simulink model "validate_emotor_start_stop"  (R2015a)
settings: Solver=ode45  StartTime=0.0  StopTime=10.0  RelTol=1e-3
settings Model: Creator=Piyush  LastModifiedBy=Piyush

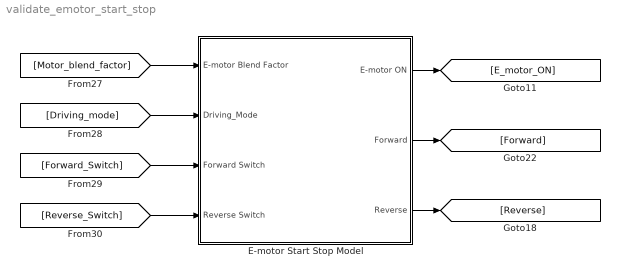
== system validate_emotor_start_stop ==
  E-motor Start Stop Model : Subsystem
  wires:
  [Motor_blend_factor] -> E-motor Start Stop Model/1(E-motor Blend Factor)
  [Driving_mode] -> E-motor Start Stop Model/2(Driving_Mode)
  [Forward_Switch] -> E-motor Start Stop Model/3(Forward Switch)
  [Reverse_Switch] -> E-motor Start Stop Model/4(Reverse Switch)
  E-motor Start Stop Model/3(Reverse) -> [Reverse]
  E-motor Start Stop Model/2(Forward) -> [Forward]
  E-motor Start Stop Model/1(E-motor ON) -> [E_motor_ON]

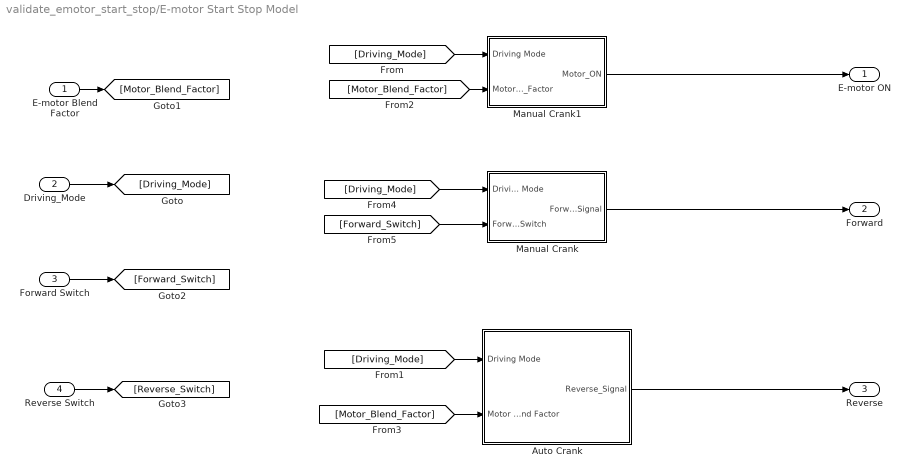
== system validate_emotor_start_stop/E-motor Start Stop Model ==
  E-motor Blend Factor : Inport
  Driving_Mode : Inport  Port=2
  Forward Switch : Inport  Port=3
  Reverse Switch : Inport  Port=4
  Auto Crank : Subsystem
  Manual Crank : Subsystem
  Manual Crank1 : Subsystem
  E-motor ON : Outport
  Forward : Outport  Port=2
  Reverse : Outport  Port=3
  wires:
  [Forward_Switch] -> Manual Crank/2(Forward Switch)
  Manual Crank1/1(Motor_ON) -> E-motor ON/1
  [Driving_Mode] -> Manual Crank1/1(Driving Mode)
  [Driving_Mode] -> Auto Crank/1(Driving Mode)
  [Motor_Blend_Factor] -> Manual Crank1/2(Motor_Blend_Factor)
  [Motor_Blend_Factor] -> Auto Crank/2(Motor Blend Factor)
  [Driving_Mode] -> Manual Crank/1(Driving Mode)
  E-motor Blend Factor/1 -> [Motor_Blend_Factor]
  Driving_Mode/1 -> [Driving_Mode]
  Forward Switch/1 -> [Forward_Switch]
  Reverse Switch/1 -> [Reverse_Switch]
  Auto Crank/1(Reverse_Signal) -> Reverse/1
  Manual Crank/1(Forward_Signal) -> Forward/1

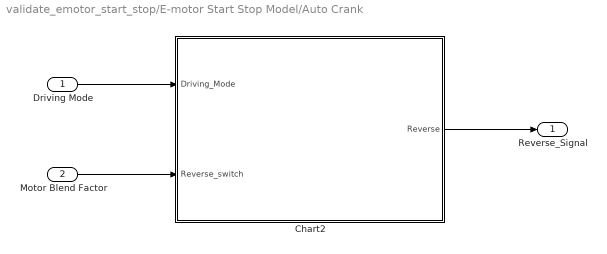
== system validate_emotor_start_stop/E-motor Start Stop Model/Auto Crank ==
  Driving Mode : Inport
  Motor Blend Factor : Inport  Port=2
  Chart2 : Stateflow chart  TreatAsAtomicUnit=on
  Reverse_Signal : Outport
  wires:
  Chart2/1(Reverse) -> Reverse_Signal/1
  Driving Mode/1 -> Chart2/1(Driving_Mode)
  Motor Blend Factor/1 -> Chart2/2(Reverse_switch)

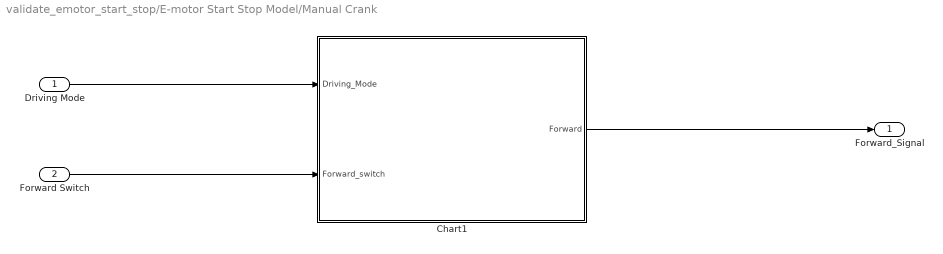
== system validate_emotor_start_stop/E-motor Start Stop Model/Manual Crank ==
  Driving Mode : Inport
  Forward Switch : Inport  Port=2
  Chart1 : Stateflow chart  TreatAsAtomicUnit=on
  Forward_Signal : Outport
  wires:
  Chart1/1(Forward) -> Forward_Signal/1
  Driving Mode/1 -> Chart1/1(Driving_Mode)
  Forward Switch/1 -> Chart1/2(Forward_switch)

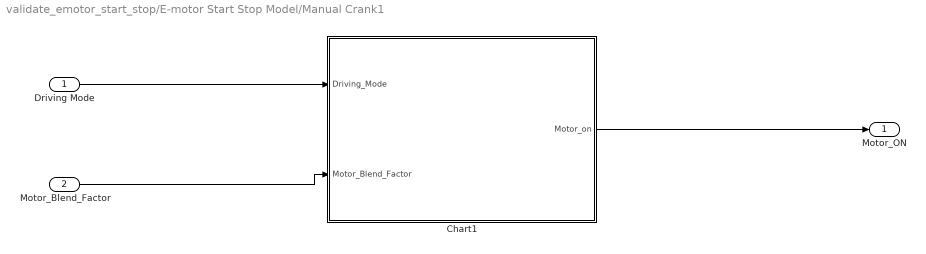
== system validate_emotor_start_stop/E-motor Start Stop Model/Manual Crank1 ==
  Driving Mode : Inport
  Motor_Blend_Factor : Inport  Port=2
  Chart1 : Stateflow chart  TreatAsAtomicUnit=on
  Motor_ON : Outport
  wires:
  Driving Mode/1 -> Chart1/1(Driving_Mode)
  Motor_Blend_Factor/1 -> Chart1/2(Motor_Blend_Factor)
  Chart1/1(Motor_on) -> Motor_ON/1

== stateflow chart validate_emotor_start_stop/E-motor Start Stop Model/Auto Crank/Chart2 ==
  state REVERSE_ON
    during: Reverse=1;
  state REVERSE_OFF
    during: Reverse=0;
  REVERSE_ON -> REVERSE_OFF : [Driving_Mode==2||Driving_Mode==3]
  REVERSE_OFF -> REVERSE_ON : [Driving_Mode==1&&Reverse_switch==1]
  (default) -> REVERSE_OFF
  data: Driving_Mode input; Reverse_switch input; Reverse output

== stateflow chart validate_emotor_start_stop/E-motor Start Stop Model/Manual Crank/Chart1 ==
  state FORWARD_ON
    during: Forward=1;
  state FORWARD_OFF
    during: Forward=0;
  FORWARD_ON -> FORWARD_OFF : [Driving_Mode==3]
  FORWARD_OFF -> FORWARD_ON [order 1] : [Driving_Mode==2]
  FORWARD_OFF -> FORWARD_ON [order 2] : [Driving_Mode==1&&Forward_switch==1]
  (default) -> FORWARD_OFF
  data: Driving_Mode input; Forward_switch input; Forward output

== stateflow chart validate_emotor_start_stop/E-motor Start Stop Model/Manual Crank1/Chart1 ==
  state MOTOR_ON
    during: Motor_on=1;
  state MOTOR_OFF
    during: Motor_on=0;
  MOTOR_ON -> MOTOR_OFF [order 2] : [Driving_Mode==2&&Motor_Blend_Factor<0.01]
  MOTOR_ON -> MOTOR_OFF [order 1] : [Driving_Mode==3]
  MOTOR_OFF -> MOTOR_ON [order 1] : [Driving_Mode==1]
  MOTOR_OFF -> MOTOR_ON [order 2] : [Driving_Mode==2&&Motor_Blend_Factor>0.01]
  (default) -> MOTOR_OFF
  data: Driving_Mode input; Motor_Blend_Factor input; Motor_on output
